simulink model "Exercise4_javi"  (R2018b)
settings: Solver=VariableStepAuto  StartTime=0.0  StopTime=1  RelTol=1e-3
undefined symbols (not defined in the file or in its folder): sigbuilder_block
libraries: arduinolib x1
settings Model: Creator=tuxtorn  LastModifiedBy=av5er

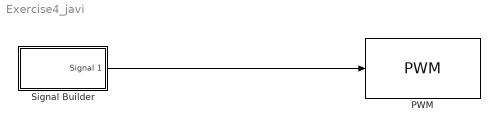
== system Exercise4_javi ==
  PWM : arduinolib/PWM  pinNumber=8  EnableInputFrequency=off  InitialFrequency=2000  InitialDutyCycle=0  NotificationType=None  blockPlatform=arduino
  Signal Builder : Subsystem  Tag=STV Subsys  LoadFcn=sigbuilder_block('load');  StartFcn=sigbuilder_block('start');  StopFcn=sigbuilder_block('stop');  ClipboardFcn=sigbuilder_block('clipboard');  mask(Sigbuilder block){tuvar=[0:10]}
      mask help: Simulink:masks:SigbuilderBlock_MD
      mask init:
      | if ~strcmp(get_param(bdroot(gcbh),'SimulationStatus'),'stopped') tuvar = sigbuilder_block('maskInit'); end
      settings: CopyFcn=sigbuilder_block('copy');  DeleteFcn=sigbuilder_block('delete');  ModelCloseFcn=sigbuilder_block('modelClose');  PreSaveFcn=sigbuilder_block('preSave');  PauseFcn=sigbuilder_block('pause');  ContinueFcn=sigbuilder_block('continue');  NameChangeFcn=sigbuilder_block('namechange');  OpenFcn=sigbuilder_block('open',[6 0 1428 711.75 ]);  CloseFcn=sigbuilder_block('close');
      mask Display: plot(0, 0, 100, 100,[2, 2, 32, 32, 2], [68, 8, 8, 68, 68],[32, 2], [38, 38], [32, 19, 2],[53, 60, 44], [32, 17, 17, 2],[16, 16, 31, 31]);txt = getActiveGroup(gcbh);text(2, 100, txt,'verticalAlignment', 'top');
  wires:
  Signal Builder/1(Signal 1) -> PWM/1

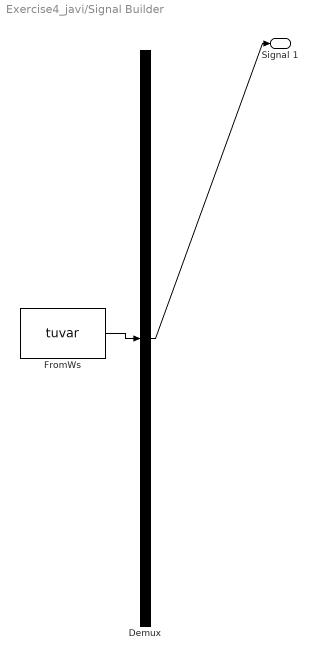
== system Exercise4_javi/Signal Builder ==
  Demux : Demux  Tag=STV Demux  Outputs=1
  FromWs : FromWorkspace  Tag=STV FromWs  VariableName=tuvar  SampleTime=0
      SigBuilderData=|
      | common.afterFinalStr = 'Extrapolate'
      | common.sampleTime = 0
      | dataSet.timeRange = [0 17.01]
      | dataSet.name = 'Group 1'
      | sbobj.Groups.Name = 'Group 1'
      | sbobj.Groups.Signals.Name = 'Signal 1'
      | sbobj.Groups.Signals.XData = [0 0.99 1 1.31 2 2 3 3 3.1764 4 4 4.2352 5 5 5.294 6 6 6.3528 7 7 7.4116 8 8 8.4704 9 9 9.5292 10 10 10.588 11 11 11.6468 12 12 12.7056 13 13 13.7644 14 14 14.8232 15 15 15.882 16 16 16.9408 17 17 17.01]
      | sbobj.Groups.Signals.YData = [0 0 0.0588 0.0588 0.0588 0.1176 0.1176 0.1764 0.1764 0.1764 0.2352 0.2352 0.2352 0.294 0.294 0.294 0.3528 0.3528 0.3528 0.4116 0.4116 0.4116 0.4704 0.4704 0.4704 0.5292 0.5292 0.5292 0.588 0.588 0.588 0.6468 0.6468 0.6468 0.7056 0.7056 0.7056 0.7644 0.7644 0.7644 0.8232 0.8232 0.8232 0.882 0.882 0.882 0.9408 0.9408 0.9408 1 1]
      | sbobj.Groups.TimeRange = [0 17.01]
  Signal 1 : Outport  Tag=STV Outport
  wires:
  FromWs/1 -> Demux/1
  Demux/1 -> Signal 1/1
